simulink model "balancing_sim_model_RL_load_Enes_parallel"  (R2018a)
settings: Solver=ode4  StartTime=0.0  StopTime=Tfinal  FixedStep=Ts  RelTol=1e-3  EnableMultiTasking=on
values from neighbouring files (symbols this model uses):
  Cdc = 15e-6    (= 1.5e-05)    [balancing_sim_parameters.m]
  Cdcrec = 2e-3    (= 0.002)    [balancing_sim_parameters.m]
  delta = 0    [balancing_sim_parameters.m]
  GridFreq = 50    [balancing_sim_parameters.m]
  Lload_1A = 36e-3    (= 0.036)    [balancing_sim_parameters.m]
  Lload_1B = 34e-3    (= 0.034)    [balancing_sim_parameters.m]
  Lload_1C = 36e-3    (= 0.036)    [balancing_sim_parameters.m]
  Lload_2A = 26e-3    (= 0.026)    [balancing_sim_parameters.m]
  Lload_2B = 26e-3    (= 0.026)    [balancing_sim_parameters.m]
  Lload_2C = 26e-3    (= 0.026)    [balancing_sim_parameters.m]
  ma1 = 0.9    [balancing_sim_parameters.m]
  ma2 = 0.9    [balancing_sim_parameters.m]
  phase = [0 90 0 90]    [balancing_sim_parameters.m]
  Rin = 70    [balancing_sim_parameters.m]
  Ripth = 0.08    [balancing_sim_parameters.m]
  Rload_1A = 15.26    [balancing_sim_parameters.m]
  Rload_1B = 15.31    [balancing_sim_parameters.m]
  Rload_1C = 15.26    [balancing_sim_parameters.m]
  Rload_2A = 14.02    [balancing_sim_parameters.m]
  Rload_2B = 14.03    [balancing_sim_parameters.m]
  Rload_2C = 14.00    (= 14)    [balancing_sim_parameters.m]
  Ts = 1e-6    (= 1e-06)    [balancing_sim_parameters.m]
  Vacrms = 230    [balancing_sim_parameters.m]
  Vin = Vdc + Rin*(Pout/Vdc)+3    (= 1061.51851852)    [balancing_sim_parameters.m]
  wout = 2*pi*fout    (= 314.159265359)    [balancing_sim_parameters.m]
undefined symbols (not defined in the file or in its folder): Lload, Rload
libraries: powerlib x45, powerlib_meascontrol x27, simulink x8
settings Model: SimulationMode=accelerator  Creator=ugurm  LastModifiedBy=enes_
settings DataIOCC: LimitDataPoints=on  SaveFormat=Array
settings OptimizationCC: LifeSpan=inf
settings DebuggingCC: UnderspecifiedInitializationDetection=Classic  MergeDetectMultiDrivingBlocksExec=none  SolverPrmCheckMsg=warning  StateNameClashWarn=warning  SFUnexpectedBacktrackingDiag=warning  SFNoUnconditionalDefaultTransitionDiag=warning  SFExecutionAtInitializationDiag=none
settings HardwareCC: ProdBitPerPointer=32  ProdBitPerSizeT=32  ProdBitPerPtrDiffT=32  ProdLargestAtomicFloat=None  ProdIntDivRoundTo=Undefined  ProdEndianess=Unspecified  ProdWordSize=32  ProdHWDeviceType=32-bit Generic
settings ModelReferenceCC: PropagateSignalLabelsOutOfModel=off
settings CodeAppCC: StateflowObjectComments=on
settings GRTTargetCC: TargetLangStandard=C89/C90 (ANSI)  GeneratePreprocessorConditionals=Disable all
settings ConfigComp: CovMetricSettings=dw  CovHtmlReporting=on  CovSaveCumulativeToWorkspaceVar=on  CovSaveSingleToWorkspaceVar=on  CovExternalEMLEnable=off
settings SimscapeCC: SimscapeNormalizeSystem=off

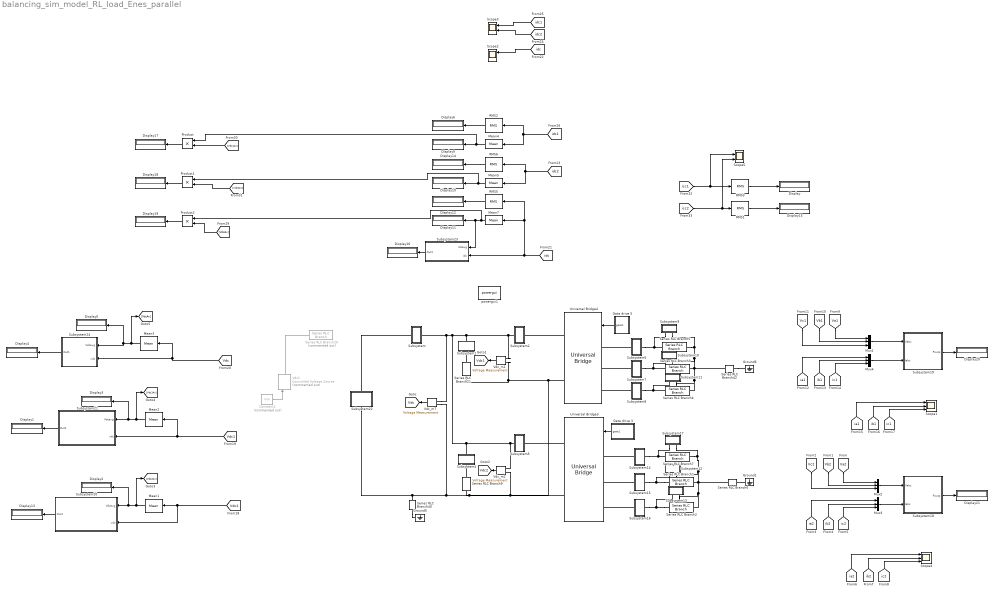
== system balancing_sim_model_RL_load_Enes_parallel ==
  Constant1 : Constant  Commented=on  Value=Vin
  Display{,1..6,9..21} (20 alike) : Display
  Gate drive 3 : Subsystem
  Gate drive 5 : Subsystem
  Ground1 : powerlib/Elements/Ground  LConnTagsString=a
  Ground5 : powerlib/Elements/Ground  LConnTagsString=a
  Ground6 : powerlib/Elements/Ground  LConnTagsString=a
  Mean{1..5,7} (6 alike) : powerlib_meascontrol/Measurements/Mean  Freq=fout  Vinit=0  Ts=0
  Mux{1..4} (4 alike) : Mux  Inputs=3
  Product : Product
  Product1 : Product
  Product2 : Product
  RMS{1..3,5..6} (5 alike) : powerlib_meascontrol/Measurements/RMS  TrueRMS=on  Freq=fout  RMSInit=0  Ts=0
  Scope1 : Scope  NumInputPorts=3
  Scope2 : Scope  NumInputPorts=2
  Scope3 : Scope  NumInputPorts=2
  Scope4 : Scope  NumInputPorts=3
  Scope5 : Scope  NumInputPorts=2
  Series RLC Branch1 : powerlib/Elements/Series RLC Branch  LConnTagsString=__new0  RConnTagsString=__new0  BranchType=RL  Resistance=Rload_2B  Inductance=Lload_2B  SetiL0=off  InitialCurrent=0  Capacitance=1e-6  Setx0=off  InitialVoltage=0  Measurements=None
  Series RLC Branch2 : powerlib/Elements/Series RLC Branch  LConnTagsString=__new0  RConnTagsString=__new0  BranchType=RL  Resistance=Rload_2C  Inductance=Lload_2C  SetiL0=off  InitialCurrent=0  Capacitance=1e-6  Setx0=off  InitialVoltage=0  Measurements=None
  Series RLC Branch20 : powerlib/Elements/Series RLC Branch  Commented=on  LConnTagsString=__new0  RConnTagsString=__new0  BranchType=R  Resistance=Rin  Inductance=1e-3  SetiL0=off  InitialCurrent=0  Capacitance=1e-6  Setx0=off  InitialVoltage=0  Measurements=None
  Series RLC Branch21 : powerlib/Elements/Series RLC Branch  LConnTagsString=__new0  RConnTagsString=__new0  BranchType=C  Resistance=Rload  Inductance=Lload  SetiL0=off  InitialCurrent=0  Capacitance=Cdc  Setx0=off  InitialVoltage=0  Measurements=None
  Series RLC Branch3 : powerlib/Elements/Series RLC Branch  LConnTagsString=__new0  RConnTagsString=__new0  BranchType=RL  Resistance=Rload_1B  Inductance=Lload_1B  SetiL0=off  InitialCurrent=0  Capacitance=1e-6  Setx0=off  InitialVoltage=0  Measurements=None
  Series RLC Branch4 : powerlib/Elements/Series RLC Branch  LConnTagsString=__new0  RConnTagsString=__new0  BranchType=RL  Resistance=Rload_1C  Inductance=Lload_1C  SetiL0=off  InitialCurrent=0  Capacitance=1e-6  Setx0=off  InitialVoltage=0  Measurements=None
  Series RLC Branch40 : powerlib/Elements/Series RLC Branch  LConnTagsString=__new0  RConnTagsString=__new0  BranchType=R  Resistance=1e12  Inductance=Lload  SetiL0=off  InitialCurrent=0  Capacitance=1e-6  Setx0=off  InitialVoltage=0  Measurements=None
  Series RLC Branch42 : powerlib/Elements/Series RLC Branch  LConnTagsString=__new0  RConnTagsString=__new0  BranchType=R  Resistance=1e12  Inductance=Lload  SetiL0=off  InitialCurrent=0  Capacitance=1e-6  Setx0=off  InitialVoltage=0  Measurements=None
  Series RLC Branch5 : powerlib/Elements/Series RLC Branch  LConnTagsString=__new0  RConnTagsString=__new0  BranchType=RL  Resistance=Rload_1A  Inductance=Lload_1A  SetiL0=off  InitialCurrent=0  Capacitance=1e-6  Setx0=off  InitialVoltage=0  Measurements=None
  Series RLC Branch6 : powerlib/Elements/Series RLC Branch  LConnTagsString=__new0  RConnTagsString=__new0  BranchType=R  Resistance=1e12  Inductance=Lload  SetiL0=off  InitialCurrent=0  Capacitance=1e-6  Setx0=off  InitialVoltage=0  Measurements=None
  Series RLC Branch7 : powerlib/Elements/Series RLC Branch  LConnTagsString=__new0  RConnTagsString=__new0  BranchType=RL  Resistance=Rload_2A  Inductance=Lload_2A  SetiL0=off  InitialCurrent=0  Capacitance=1e-6  Setx0=off  InitialVoltage=0  Measurements=None
  Series RLC Branch9 : powerlib/Elements/Series RLC Branch  LConnTagsString=__new0  RConnTagsString=__new0  BranchType=C  Resistance=Rload  Inductance=Lload  SetiL0=off  InitialCurrent=0  Capacitance=Cdc  Setx0=off  InitialVoltage=0  Measurements=None
  Subsystem : Subsystem
  Subsystem1 : Subsystem
  Subsystem10 : Subsystem
  Subsystem11 : Subsystem
  Subsystem12 : Subsystem
  Subsystem13 : Subsystem
  Subsystem14 : Subsystem
  Subsystem15 : Subsystem
  Subsystem16 : Subsystem
  Subsystem17 : Subsystem
  Subsystem18 : Subsystem
  Subsystem19 : Subsystem
  Subsystem2 : Subsystem
  Subsystem20 : Subsystem
  Subsystem21 : Subsystem
  Subsystem22 : Subsystem
  Subsystem23 : Subsystem
  Subsystem24 : Subsystem
  Subsystem4 : Subsystem
  Subsystem5 : Subsystem
  Subsystem6 : Subsystem
  Subsystem7 : Subsystem
  Subsystem8 : Subsystem
  Subsystem9 : Subsystem
  Universal Bridge3 : powerlib/Power Electronics/Universal Bridge  Arms=3  SnubberResistance=1e5  SnubberCapacitance=inf  Device=IGBT / Diodes  Ron=1e-6  Lon=0  ForwardVoltages="[  0  0  ]"  ForwardVoltage=0  GTOparameters=[ 10e-6 , 20e-6 ]  IGBTparameters=[0,0]  Measurements=None  Measurements_2=None  converterType=Rectifier
  Universal Bridge4 : powerlib/Power Electronics/Universal Bridge  Arms=3  SnubberResistance=1e5  SnubberCapacitance=inf  Device=IGBT / Diodes  Ron=1e-6  Lon=0  ForwardVoltages="[  0  0  ]"  ForwardVoltage=0  GTOparameters=[ 10e-6 , 20e-6 ]  IGBTparameters=[0,0]  Measurements=None  Measurements_2=None  converterType=Rectifier
  Vdc1 : powerlib/Electrical Sources/Controlled Voltage Source  Commented=on  Initialize=off  Source_Type=DC  Amplitude=200  Phase=0  Frequency=0  Measurements=None
  Vdc_m1 : powerlib/Measurements/Voltage Measurement  PhasorSimulation=off  OutputType=Complex  PSBequivalent=0
  Vdc_m2 : powerlib/Measurements/Voltage Measurement  PhasorSimulation=off  OutputType=Complex  PSBequivalent=0
  Vdc_m7 : powerlib/Measurements/Voltage Measurement  PhasorSimulation=off  OutputType=Complex  PSBequivalent=0
  powergui1 : powerlib/powergui  Priority=1  SimulationMode=Discrete  SampleTime=Ts  frequency=60  Iterations=50  frequencyindice=0  Pbase=100e6  ErrMax=1e-4  UnitsV=kV  UnitsW=MW  buscounter=0  FunctionMessages=off  echomessages=off  EnableUseOfTLC=off  CurrentSourceSwitches=off  DisableSnubberDevices=off  DisableRonSwitches=off  DisableVfSwitches=off  DisplayEquations=off  SolverType=Tustin  Interpol=off  ExternalGateDelay=off  methode=off  Ts=0  x0status=blocks  SPID=off  SwTol=0  HookPort=off  RestoreLinks=warning  ResistiveCurrentMeasurement=off  Frange=[0:2:500]  Ylog=off  Xlog=on  ShowGrid=off  save=off  variable=ZData  structure=Vdc  ZoomFFT=off  StartTime=0.04  cycles=5  DisplayStyle=5  fundamental=50  FreqAxis=off  MaxFrequency=30000  frequencyindicesteady=1  RmsSteady=1  display=off
  tag scope: Vdc1=global, Vdc2=global, Vdc=global
  wires:
  Constant1/1 -> Vdc1/1
  Vdc_m7/1 -> [Vdc]
  Vdc_m1/1 -> [Vdc1]
  Gate drive 5/1(gate1) -> Universal Bridge4/1
  Vdc_m2/1 -> [Vdc2]
  Gate drive 3/1(gate1) -> Universal Bridge3/1
  Mux3/1 -> Subsystem18/2(Iabc)
  Mux2/1 -> Subsystem18/1(Vabc)
  Subsystem18/1(Poutp) -> Display21/1
  [Va2] -> Mux2/1
  [Vb2] -> Mux2/2
  [Vc2] -> Mux2/3
  [ia2] -> Mux3/1
  [ib2] -> Mux3/2
  [ic2] -> Mux3/3
  [ia2] -> Scope4/1
  [ib2] -> Scope4/2
  [ic2] -> Scope4/3
  Subsystem19/1(Poutp) -> Display20/1
  [ic1] -> Mux4/3
  Mux4/1 -> Subsystem19/2(Iabc)
  Mux1/1 -> Subsystem19/1(Vabc)
  [ia1] -> Mux4/1
  [ib1] -> Mux4/2
  [Va1] -> Mux1/1
  [Vb1] -> Mux1/2
  [Vc1] -> Mux1/3
  [ib1] -> Scope1/2
  [ic1] -> Scope1/3
  [ia1] -> Scope1/1
  Subsystem20/1(Out1) -> Display13/1
  Mean1/1 -> [Vdc2Av], Subsystem20/1(Vdcavg), Display2/1
  [Vdc2] -> Subsystem20/2(vdc), Mean1/1
  Subsystem21/1(Out1) -> Display1/1
  [Vdc1] -> Subsystem21/2(vdc), Mean2/1
  Mean2/1 -> [Vdc1Av], Subsystem21/1(Vdcavg), Display3/1
  Subsystem24/1(Out1) -> Display4/1
  [Vdc] -> Subsystem24/2(vdc), Mean3/1
  RMS2/1 -> Display6/1
  RMS5/1 -> Display12/1
  RMS6/1 -> Display14/1
  Subsystem23/1(Out1) -> Display16/1
  [idc] -> Mean7/1, RMS5/1, Subsystem23/2(idc)
  [idc] -> Scope2/1
  [idc2] -> Mean5/1, RMS6/1
  [idc2] -> Scope3/2
  [idc1] -> Scope3/1
  [idc1] -> RMS2/1, Mean4/1
  Mean7/1 -> Product2/1, Subsystem23/1(Idcavg), Display11/1
  Mean5/1 -> Product1/1, Display10/1
  Product1/1 -> Display18/1
  Product/1 -> Display17/1
  Mean4/1 -> Product/1, Display9/1
  Product2/1 -> Display19/1
  [VdcAv] -> Product2/2
  [Vdc1Av] -> Product/2
  [Vdc2Av] -> Product1/2
  RMS3/1 -> Display/1
  RMS1/1 -> Display15/1
  [icc1] -> Scope5/1, RMS3/1
  [icc2] -> Scope5/2, RMS1/1
  Mean3/1 -> [VdcAv], Subsystem24/1(Vdcavg), Display5/1
  connections:
  Series RLC Branch40/RConn1 -- Ground5/LConn1
  Vdc1/RConn1 -- Series RLC Branch20/LConn1
  Series RLC Branch21/LConn1 -- Subsystem1/LConn1
  Vdc_m2/LConn2 -- Universal Bridge3/RConn2 -- Subsystem22/LConn1 -- Series RLC Branch40/LConn1 -- Vdc_m7/LConn2 -- Universal Bridge4/RConn2 -- Series RLC Branch21/RConn1 -- Vdc_m1/LConn2 -- Series RLC Branch9/RConn1
  Universal Bridge4/RConn1 -- Subsystem2/RConn1
  Series RLC Branch9/LConn1 -- Subsystem4/LConn1
  Vdc_m7/LConn1 -- Vdc_m1/LConn1 -- Subsystem2/LConn1 -- Subsystem1/RConn1 -- Subsystem5/LConn1 -- Vdc_m2/LConn1 -- Subsystem4/RConn1 -- Subsystem/RConn1
  Universal Bridge3/RConn1 -- Subsystem5/RConn1
  Subsystem6/LConn1 -- Universal Bridge4/LConn1
  Subsystem8/LConn1 -- Universal Bridge4/LConn3
  Subsystem7/LConn1 -- Universal Bridge4/LConn2
  Subsystem8/RConn1 -- Subsystem11/LConn1 -- Series RLC Branch4/LConn1
  Subsystem7/RConn1 -- Subsystem10/LConn1 -- Series RLC Branch3/LConn1
  Series RLC Branch5/RConn1 -- Subsystem9/LConn2 -- Subsystem10/LConn2 -- Subsystem11/LConn2 -- Series RLC Branch4/RConn1 -- Series RLC Branch3/RConn1 -- Series RLC Branch42/LConn1
  Series RLC Branch42/RConn1 -- Ground6/LConn1
  Subsystem6/RConn1 -- Subsystem9/LConn1 -- Series RLC Branch5/LConn1
  Series RLC Branch2/RConn1 -- Subsystem13/LConn2 -- Subsystem17/LConn2 -- Series RLC Branch7/RConn1 -- Subsystem12/LConn2 -- Series RLC Branch1/RConn1 -- Series RLC Branch6/LConn1
  Subsystem17/LConn1 -- Series RLC Branch7/LConn1 -- Subsystem14/RConn1
  Series RLC Branch2/LConn1 -- Subsystem13/LConn1 -- Subsystem16/RConn1
  Series RLC Branch1/LConn1 -- Subsystem15/RConn1 -- Subsystem12/LConn1
  Subsystem14/LConn1 -- Universal Bridge3/LConn1
  Subsystem15/LConn1 -- Universal Bridge3/LConn2
  Subsystem16/LConn1 -- Universal Bridge3/LConn3
  Ground1/LConn1 -- Series RLC Branch6/RConn1
  Subsystem22/RConn1 -- Subsystem/LConn1

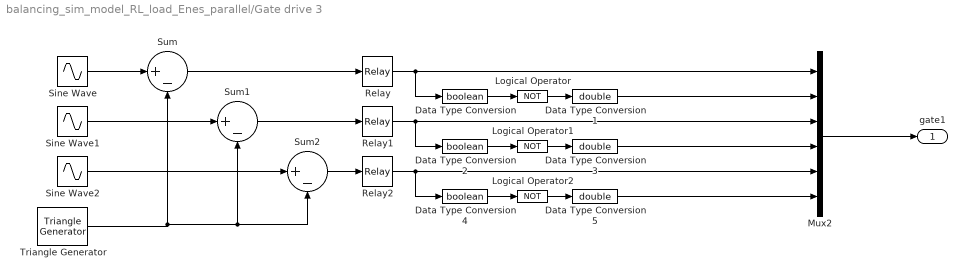
== system balancing_sim_model_RL_load_Enes_parallel/Gate drive 3 ==
  Data Type Conversion : DataTypeConversion  OutDataTypeStr=boolean
  Data Type Conversion1 : DataTypeConversion  OutDataTypeStr=double
  Data Type Conversion2 : DataTypeConversion  OutDataTypeStr=boolean
  Data Type Conversion3 : DataTypeConversion  OutDataTypeStr=double
  Data Type Conversion4 : DataTypeConversion  OutDataTypeStr=boolean
  Data Type Conversion5 : DataTypeConversion  OutDataTypeStr=double
  Logical Operator : Logic  Operator=NOT  AllPortsSameDT=off  OutDataTypeStr=boolean
  Logical Operator1 : Logic  Operator=NOT  AllPortsSameDT=off  OutDataTypeStr=boolean
  Logical Operator2 : Logic  Operator=NOT  AllPortsSameDT=off  OutDataTypeStr=boolean
  Mux2 : Mux  Inputs=6
  Relay : Relay
  Relay1 : Relay
  Relay2 : Relay
  Sine Wave : Sin  Amplitude=ma2  Frequency=wout  Phase=delta  SampleTime=0
  Sine Wave1 : Sin  Amplitude=ma2  Frequency=wout  Phase=-2*pi/3+delta  SampleTime=0
  Sine Wave2 : Sin  Amplitude=ma2  Frequency=wout  Phase=2*pi/3+delta  SampleTime=0
  Sum : Sum  Inputs=|+-
  Sum1 : Sum  Inputs=|+-
  Sum2 : Sum  Inputs=|+-
  Triangle Generator : powerlib_meascontrol/Pulse & Signal Generators/Triangle Generator  Freq=fsw  Phase=phase(3)  Ts=Ts
  gate1 : Outport
  wires:
  Sine Wave/1 -> Sum/1
  Triangle Generator/1 -> Sum1/2, Sum2/2, Sum/2
  Sine Wave1/1 -> Sum1/1
  Sine Wave2/1 -> Sum2/1
  Sum/1 -> Relay/1
  Sum1/1 -> Relay1/1
  Sum2/1 -> Relay2/1
  Data Type Conversion/1 -> Logical Operator/1
  Relay/1 -> Data Type Conversion/1, Mux2/1
  Logical Operator/1 -> Data Type Conversion1/1
  Data Type Conversion1/1 -> Mux2/2
  Data Type Conversion2/1 -> Logical Operator1/1
  Relay1/1 -> Data Type Conversion2/1, Mux2/3
  Logical Operator1/1 -> Data Type Conversion3/1
  Data Type Conversion3/1 -> Mux2/4
  Data Type Conversion4/1 -> Logical Operator2/1
  Relay2/1 -> Data Type Conversion4/1, Mux2/5
  Logical Operator2/1 -> Data Type Conversion5/1
  Data Type Conversion5/1 -> Mux2/6
  Mux2/1 -> gate1/1

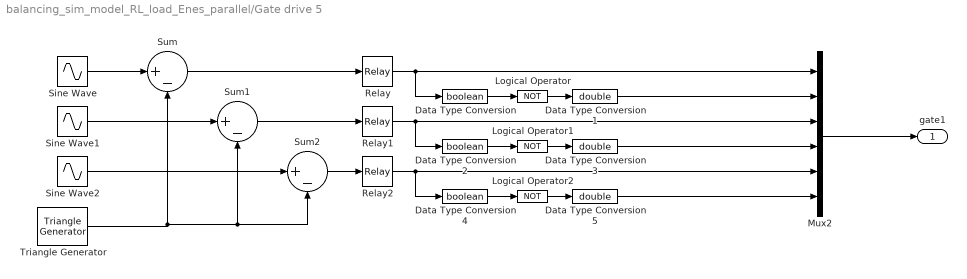
== system balancing_sim_model_RL_load_Enes_parallel/Gate drive 5 ==
  Data Type Conversion : DataTypeConversion  OutDataTypeStr=boolean
  Data Type Conversion1 : DataTypeConversion  OutDataTypeStr=double
  Data Type Conversion2 : DataTypeConversion  OutDataTypeStr=boolean
  Data Type Conversion3 : DataTypeConversion  OutDataTypeStr=double
  Data Type Conversion4 : DataTypeConversion  OutDataTypeStr=boolean
  Data Type Conversion5 : DataTypeConversion  OutDataTypeStr=double
  Logical Operator : Logic  Operator=NOT  AllPortsSameDT=off  OutDataTypeStr=boolean
  Logical Operator1 : Logic  Operator=NOT  AllPortsSameDT=off  OutDataTypeStr=boolean
  Logical Operator2 : Logic  Operator=NOT  AllPortsSameDT=off  OutDataTypeStr=boolean
  Mux2 : Mux  Inputs=6
  Relay : Relay
  Relay1 : Relay
  Relay2 : Relay
  Sine Wave : Sin  Amplitude=ma1  Frequency=wout  Phase=delta  SampleTime=0
  Sine Wave1 : Sin  Amplitude=ma1  Frequency=wout  Phase=-2*pi/3+delta  SampleTime=0
  Sine Wave2 : Sin  Amplitude=ma1  Frequency=wout  Phase=2*pi/3+delta  SampleTime=0
  Sum : Sum  Inputs=|+-
  Sum1 : Sum  Inputs=|+-
  Sum2 : Sum  Inputs=|+-
  Triangle Generator : powerlib_meascontrol/Pulse & Signal Generators/Triangle Generator  Freq=fsw  Phase=phase(1)  Ts=Ts
  gate1 : Outport
  wires:
  Sine Wave/1 -> Sum/1
  Triangle Generator/1 -> Sum1/2, Sum2/2, Sum/2
  Sine Wave1/1 -> Sum1/1
  Sine Wave2/1 -> Sum2/1
  Sum/1 -> Relay/1
  Sum1/1 -> Relay1/1
  Sum2/1 -> Relay2/1
  Data Type Conversion/1 -> Logical Operator/1
  Relay/1 -> Data Type Conversion/1, Mux2/1
  Logical Operator/1 -> Data Type Conversion1/1
  Data Type Conversion1/1 -> Mux2/2
  Data Type Conversion2/1 -> Logical Operator1/1
  Relay1/1 -> Data Type Conversion2/1, Mux2/3
  Logical Operator1/1 -> Data Type Conversion3/1
  Data Type Conversion3/1 -> Mux2/4
  Data Type Conversion4/1 -> Logical Operator2/1
  Relay2/1 -> Data Type Conversion4/1, Mux2/5
  Logical Operator2/1 -> Data Type Conversion5/1
  Data Type Conversion5/1 -> Mux2/6
  Mux2/1 -> gate1/1

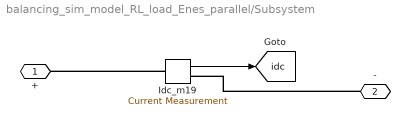
== system balancing_sim_model_RL_load_Enes_parallel/Subsystem ==
  Idc_m19 : powerlib/Measurements/Current Measurement  PhasorSimulation=off  OutputType=Complex  PSBequivalent=0
  + : PMIOPort  Side=Left
  " -" : PMIOPort  Port=2  Side=Right
  tag scope: idc=global
  wires:
  Idc_m19/1 -> [idc]
  connections:
  " -"/RConn1 -- Idc_m19/RConn1
  Idc_m19/LConn1 -- +/RConn1

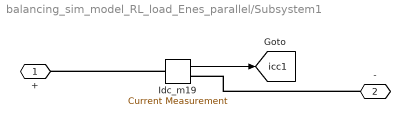
== system balancing_sim_model_RL_load_Enes_parallel/Subsystem1 ==
  Idc_m19 : powerlib/Measurements/Current Measurement  PhasorSimulation=off  OutputType=Complex  PSBequivalent=0
  + : PMIOPort  Side=Left
  " -" : PMIOPort  Port=2  Side=Right
  tag scope: icc1=global
  wires:
  Idc_m19/1 -> [icc1]
  connections:
  " -"/RConn1 -- Idc_m19/RConn1
  Idc_m19/LConn1 -- +/RConn1

== system balancing_sim_model_RL_load_Enes_parallel/Subsystem10 ==
  Vdc_m3 : powerlib/Measurements/Voltage Measurement  PhasorSimulation=off  OutputType=Complex  PSBequivalent=0
  + : PMIOPort  Side=Left
  - : PMIOPort  Port=2  Side=Left
  tag scope: Vb1=global
  wires:
  Vdc_m3/1 -> [Vb1]
  connections:
  Vdc_m3/LConn1 -- +/RConn1
  Vdc_m3/LConn2 -- -/RConn1

== system balancing_sim_model_RL_load_Enes_parallel/Subsystem11 ==
  Vdc_m3 : powerlib/Measurements/Voltage Measurement  PhasorSimulation=off  OutputType=Complex  PSBequivalent=0
  + : PMIOPort  Side=Left
  - : PMIOPort  Port=2  Side=Left
  tag scope: Vc1=global
  wires:
  Vdc_m3/1 -> [Vc1]
  connections:
  Vdc_m3/LConn1 -- +/RConn1
  Vdc_m3/LConn2 -- -/RConn1

== system balancing_sim_model_RL_load_Enes_parallel/Subsystem12 ==
  Vdc_m3 : powerlib/Measurements/Voltage Measurement  PhasorSimulation=off  OutputType=Complex  PSBequivalent=0
  + : PMIOPort  Side=Left
  - : PMIOPort  Port=2  Side=Left
  tag scope: Vb2=global
  wires:
  Vdc_m3/1 -> [Vb2]
  connections:
  Vdc_m3/LConn1 -- +/RConn1
  Vdc_m3/LConn2 -- -/RConn1

== system balancing_sim_model_RL_load_Enes_parallel/Subsystem13 ==
  Vdc_m3 : powerlib/Measurements/Voltage Measurement  PhasorSimulation=off  OutputType=Complex  PSBequivalent=0
  + : PMIOPort  Side=Left
  - : PMIOPort  Port=2  Side=Left
  tag scope: Vc2=global
  wires:
  Vdc_m3/1 -> [Vc2]
  connections:
  Vdc_m3/LConn1 -- +/RConn1
  Vdc_m3/LConn2 -- -/RConn1

== system balancing_sim_model_RL_load_Enes_parallel/Subsystem14 ==
  Idc_m19 : powerlib/Measurements/Current Measurement  PhasorSimulation=off  OutputType=Complex  PSBequivalent=0
  + : PMIOPort  Side=Left
  " -" : PMIOPort  Port=2  Side=Right
  tag scope: ia2=global
  wires:
  Idc_m19/1 -> [ia2]
  connections:
  " -"/RConn1 -- Idc_m19/RConn1
  Idc_m19/LConn1 -- +/RConn1

== system balancing_sim_model_RL_load_Enes_parallel/Subsystem15 ==
  Idc_m19 : powerlib/Measurements/Current Measurement  PhasorSimulation=off  OutputType=Complex  PSBequivalent=0
  + : PMIOPort  Side=Left
  " -" : PMIOPort  Port=2  Side=Right
  tag scope: ib2=global
  wires:
  Idc_m19/1 -> [ib2]
  connections:
  " -"/RConn1 -- Idc_m19/RConn1
  Idc_m19/LConn1 -- +/RConn1

== system balancing_sim_model_RL_load_Enes_parallel/Subsystem16 ==
  Idc_m19 : powerlib/Measurements/Current Measurement  PhasorSimulation=off  OutputType=Complex  PSBequivalent=0
  + : PMIOPort  Side=Left
  " -" : PMIOPort  Port=2  Side=Right
  tag scope: ic2=global
  wires:
  Idc_m19/1 -> [ic2]
  connections:
  " -"/RConn1 -- Idc_m19/RConn1
  Idc_m19/LConn1 -- +/RConn1

== system balancing_sim_model_RL_load_Enes_parallel/Subsystem17 ==
  Vdc_m3 : powerlib/Measurements/Voltage Measurement  PhasorSimulation=off  OutputType=Complex  PSBequivalent=0
  + : PMIOPort  Side=Left
  - : PMIOPort  Port=2  Side=Left
  tag scope: Va2=global
  wires:
  Vdc_m3/1 -> [Va2]
  connections:
  Vdc_m3/LConn1 -- +/RConn1
  Vdc_m3/LConn2 -- -/RConn1

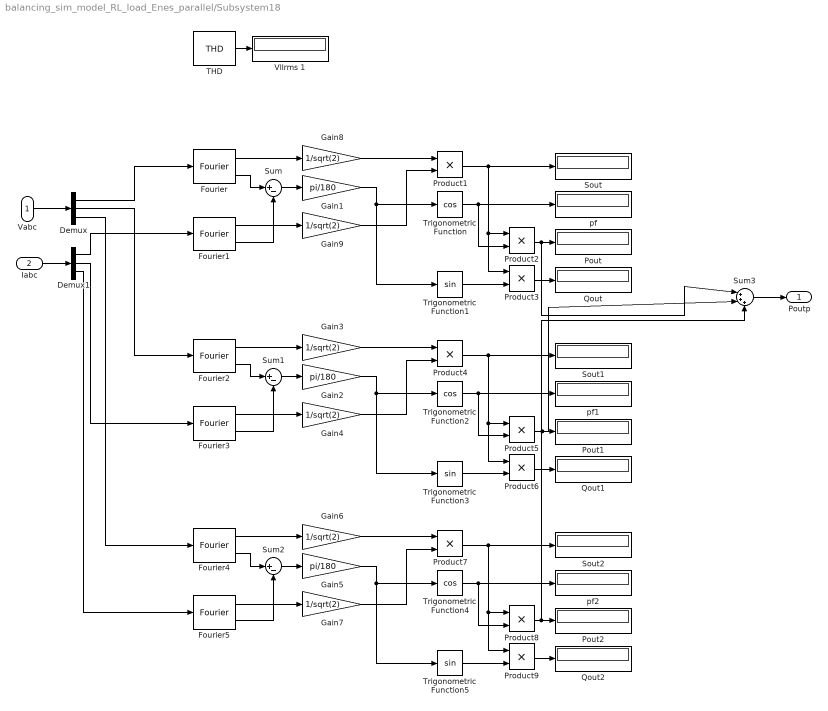
== system balancing_sim_model_RL_load_Enes_parallel/Subsystem18 ==
  Vabc : Inport
  Iabc : Inport  Port=2
  Demux : Demux  Outputs=3
  Demux1 : Demux  Outputs=3
  Fourier{,1..5} (6 alike) : powerlib_meascontrol/Measurements/Fourier  Freq=fout  n=1  InInit=[0, 0]  Ts=Ts
      settings: SourceProductName=Simscape Power Systems
  Gain1 : Gain  Gain=pi/180
  Gain2 : Gain  Gain=pi/180
  Gain{3..4,6..9} (6 alike) : Gain  Gain=1/sqrt(2)
  Gain5 : Gain  Gain=pi/180
  Pout : Display
  Pout1 : Display
  Pout2 : Display
  Product{1..9} (9 alike) : Product
  Qout : Display
  Qout1 : Display
  Qout2 : Display
  Sout : Display
      settings: Format=short_e
  Sout1 : Display
      settings: Format=short_e
  Sout2 : Display
      settings: Format=short_e
  Sum : Sum  Inputs=|+-
  Sum1 : Sum  Inputs=|+-
  Sum2 : Sum  Inputs=|+-
  Sum3 : Sum  Inputs=|+++
  THD : powerlib_meascontrol/Measurements/THD  Freq=fout  Ts=0
  Trigonometric Function : Trigonometry  Operator=cos
  Trigonometric Function1 : Trigonometry
  Trigonometric Function2 : Trigonometry  Operator=cos
  Trigonometric Function3 : Trigonometry
  Trigonometric Function4 : Trigonometry  Operator=cos
  Trigonometric Function5 : Trigonometry
  Vllrms 1 : Display
  pf : Display
  pf1 : Display
  pf2 : Display
  Poutp : Outport
  wires:
  Gain8/1 -> Product1/1
  Gain9/1 -> Product1/2
  Fourier1/1 -> Gain9/1
  Fourier/1 -> Gain8/1
  Product1/1 -> Product3/1, Product2/1, Sout/1
  Sum/1 -> Gain1/1
  Trigonometric Function/1 -> Product2/2, pf/1
  Gain1/1 -> Trigonometric Function1/1, Trigonometric Function/1
  Product2/1 -> Sum3/1, Pout/1
  THD/1 -> Vllrms 1/1
  Vabc/1 -> Demux/1
  Iabc/1 -> Demux1/1
  Fourier/2 -> Sum/1
  Fourier1/2 -> Sum/2
  Trigonometric Function1/1 -> Product3/2
  Product3/1 -> Qout/1
  Gain3/1 -> Product4/1
  Gain4/1 -> Product4/2
  Fourier3/1 -> Gain4/1
  Fourier2/1 -> Gain3/1
  Product4/1 -> Product6/1, Product5/1, Sout1/1
  Sum1/1 -> Gain2/1
  Trigonometric Function2/1 -> Product5/2, pf1/1
  Gain2/1 -> Trigonometric Function3/1, Trigonometric Function2/1
  Product5/1 -> Sum3/2, Pout1/1
  Fourier2/2 -> Sum1/1
  Fourier3/2 -> Sum1/2
  Trigonometric Function3/1 -> Product6/2
  Product6/1 -> Qout1/1
  Gain6/1 -> Product7/1
  Gain7/1 -> Product7/2
  Fourier5/1 -> Gain7/1
  Fourier4/1 -> Gain6/1
  Product7/1 -> Product9/1, Product8/1, Sout2/1
  Sum2/1 -> Gain5/1
  Trigonometric Function4/1 -> Product8/2, pf2/1
  Gain5/1 -> Trigonometric Function5/1, Trigonometric Function4/1
  Fourier4/2 -> Sum2/1
  Fourier5/2 -> Sum2/2
  Trigonometric Function5/1 -> Product9/2
  Product9/1 -> Qout2/1
  Product8/1 -> Sum3/3, Pout2/1
  Sum3/1 -> Poutp/1
  Demux/1 -> Fourier/1
  Demux/2 -> Fourier2/1
  Demux/3 -> Fourier4/1
  Demux1/1 -> Fourier1/1
  Demux1/2 -> Fourier3/1
  Demux1/3 -> Fourier5/1

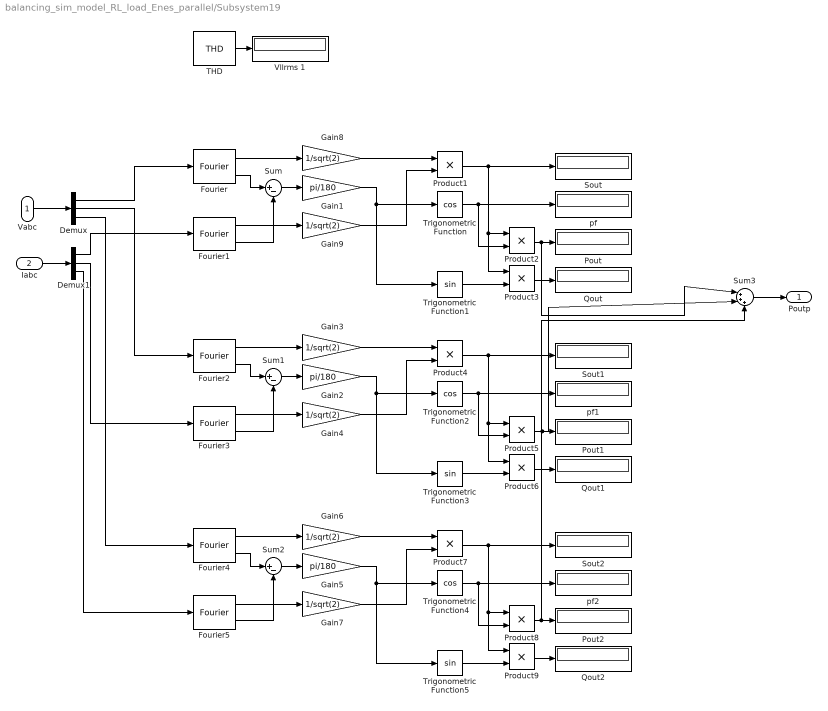
== system balancing_sim_model_RL_load_Enes_parallel/Subsystem19 ==
  Vabc : Inport
  Iabc : Inport  Port=2
  Demux : Demux  Outputs=3
  Demux1 : Demux  Outputs=3
  Fourier{,1..5} (6 alike) : powerlib_meascontrol/Measurements/Fourier  Freq=fout  n=1  InInit=[0, 0]  Ts=Ts
      settings: SourceProductName=Simscape Power Systems
  Gain1 : Gain  Gain=pi/180
  Gain2 : Gain  Gain=pi/180
  Gain{3..4,6..9} (6 alike) : Gain  Gain=1/sqrt(2)
  Gain5 : Gain  Gain=pi/180
  Pout : Display
  Pout1 : Display
  Pout2 : Display
  Product{1..9} (9 alike) : Product
  Qout : Display
  Qout1 : Display
  Qout2 : Display
  Sout : Display
      settings: Format=short_e
  Sout1 : Display
      settings: Format=short_e
  Sout2 : Display
      settings: Format=short_e
  Sum : Sum  Inputs=|+-
  Sum1 : Sum  Inputs=|+-
  Sum2 : Sum  Inputs=|+-
  Sum3 : Sum  Inputs=|+++
  THD : powerlib_meascontrol/Measurements/THD  Freq=fout  Ts=0
  Trigonometric Function : Trigonometry  Operator=cos
  Trigonometric Function1 : Trigonometry
  Trigonometric Function2 : Trigonometry  Operator=cos
  Trigonometric Function3 : Trigonometry
  Trigonometric Function4 : Trigonometry  Operator=cos
  Trigonometric Function5 : Trigonometry
  Vllrms 1 : Display
  pf : Display
  pf1 : Display
  pf2 : Display
  Poutp : Outport
  wires:
  Gain8/1 -> Product1/1
  Gain9/1 -> Product1/2
  Fourier1/1 -> Gain9/1
  Fourier/1 -> Gain8/1
  Product1/1 -> Product3/1, Product2/1, Sout/1
  Sum/1 -> Gain1/1
  Trigonometric Function/1 -> Product2/2, pf/1
  Gain1/1 -> Trigonometric Function1/1, Trigonometric Function/1
  Product2/1 -> Sum3/1, Pout/1
  THD/1 -> Vllrms 1/1
  Vabc/1 -> Demux/1
  Iabc/1 -> Demux1/1
  Fourier/2 -> Sum/1
  Fourier1/2 -> Sum/2
  Trigonometric Function1/1 -> Product3/2
  Product3/1 -> Qout/1
  Gain3/1 -> Product4/1
  Gain4/1 -> Product4/2
  Fourier3/1 -> Gain4/1
  Fourier2/1 -> Gain3/1
  Product4/1 -> Product6/1, Product5/1, Sout1/1
  Sum1/1 -> Gain2/1
  Trigonometric Function2/1 -> Product5/2, pf1/1
  Gain2/1 -> Trigonometric Function3/1, Trigonometric Function2/1
  Product5/1 -> Sum3/2, Pout1/1
  Fourier2/2 -> Sum1/1
  Fourier3/2 -> Sum1/2
  Trigonometric Function3/1 -> Product6/2
  Product6/1 -> Qout1/1
  Gain6/1 -> Product7/1
  Gain7/1 -> Product7/2
  Fourier5/1 -> Gain7/1
  Fourier4/1 -> Gain6/1
  Product7/1 -> Product9/1, Product8/1, Sout2/1
  Sum2/1 -> Gain5/1
  Trigonometric Function4/1 -> Product8/2, pf2/1
  Gain5/1 -> Trigonometric Function5/1, Trigonometric Function4/1
  Fourier4/2 -> Sum2/1
  Fourier5/2 -> Sum2/2
  Trigonometric Function5/1 -> Product9/2
  Product9/1 -> Qout2/1
  Product8/1 -> Sum3/3, Pout2/1
  Sum3/1 -> Poutp/1
  Demux/1 -> Fourier/1
  Demux/2 -> Fourier2/1
  Demux/3 -> Fourier4/1
  Demux1/1 -> Fourier1/1
  Demux1/2 -> Fourier3/1
  Demux1/3 -> Fourier5/1

== system balancing_sim_model_RL_load_Enes_parallel/Subsystem2 ==
  Idc_m19 : powerlib/Measurements/Current Measurement  PhasorSimulation=off  OutputType=Complex  PSBequivalent=0
  + : PMIOPort  Side=Left
  " -" : PMIOPort  Port=2  Side=Right
  tag scope: idc1=global
  wires:
  Idc_m19/1 -> [idc1]
  connections:
  " -"/RConn1 -- Idc_m19/RConn1
  Idc_m19/LConn1 -- +/RConn1

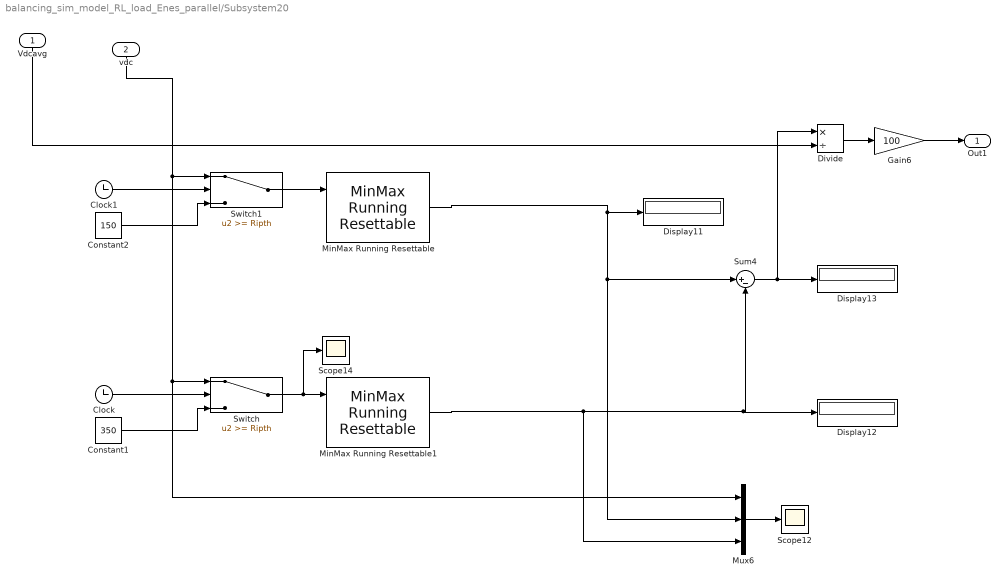
== system balancing_sim_model_RL_load_Enes_parallel/Subsystem20 ==
  Vdcavg : Inport
  vdc : Inport  Port=2
  Clock : Clock
  Clock1 : Clock
  Constant1 : Constant  Value=350  SampleTime=Ts
  Constant2 : Constant  Value=150  SampleTime=Ts
  Display11 : Display
  Display12 : Display
  Display13 : Display
  Divide : Product  Inputs=*/
  Gain6 : Gain  Gain=100
  MinMax Running Resettable : simulink/Math Operations/MinMax Running Resettable  Function=max  vinit=0.0
  MinMax Running Resettable1 : simulink/Math Operations/MinMax Running Resettable  Function=min  vinit=700
  Mux6 : Mux  Inputs=3
  Scope12 : Scope
  Scope14 : Scope
  Sum4 : Sum  Inputs=|+-
  Switch : Switch  Threshold=Ripth
  Switch1 : Switch  Threshold=Ripth
  Out1 : Outport
  wires:
  MinMax Running Resettable/1 -> Display11/1, Mux6/2, Sum4/1
  Clock/1 -> Switch/2
  Gain6/1 -> Out1/1
  Constant1/1 -> Switch/3
  MinMax Running Resettable1/1 -> Mux6/3, Display12/1, Sum4/2
  Switch/1 -> Scope14/1, MinMax Running Resettable1/1
  Sum4/1 -> Divide/1, Display13/1
  Divide/1 -> Gain6/1
  Mux6/1 -> Scope12/1
  Vdcavg/1 -> Divide/2
  vdc/1 -> Switch1/1, Mux6/1, Switch/1
  Switch1/1 -> MinMax Running Resettable/1
  Clock1/1 -> Switch1/2
  Constant2/1 -> Switch1/3

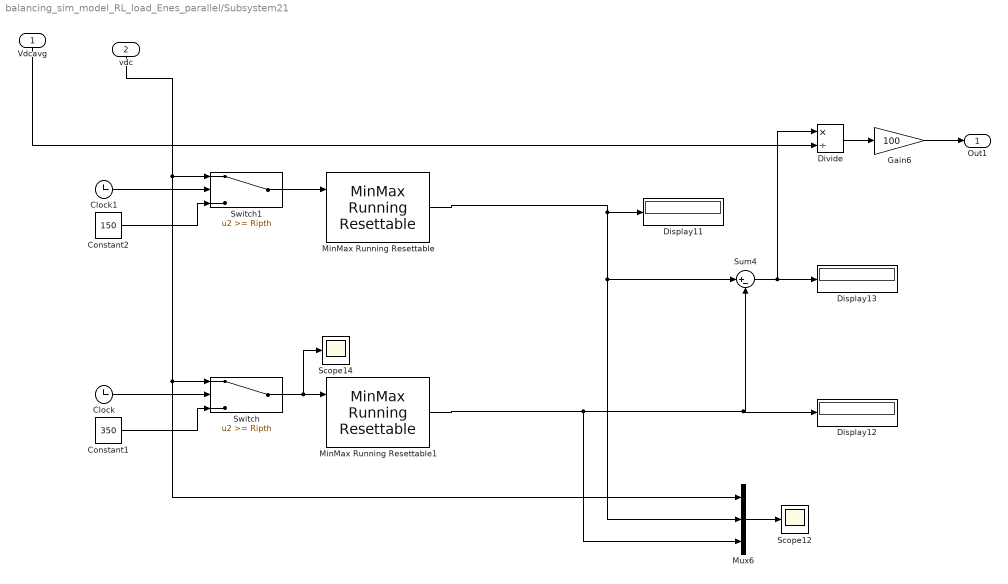
== system balancing_sim_model_RL_load_Enes_parallel/Subsystem21 ==
  Vdcavg : Inport
  vdc : Inport  Port=2
  Clock : Clock
  Clock1 : Clock
  Constant1 : Constant  Value=350  SampleTime=Ts
  Constant2 : Constant  Value=150  SampleTime=Ts
  Display11 : Display
  Display12 : Display
  Display13 : Display
  Divide : Product  Inputs=*/
  Gain6 : Gain  Gain=100
  MinMax Running Resettable : simulink/Math Operations/MinMax Running Resettable  Function=max  vinit=0.0
  MinMax Running Resettable1 : simulink/Math Operations/MinMax Running Resettable  Function=min  vinit=700
  Mux6 : Mux  Inputs=3
  Scope12 : Scope
  Scope14 : Scope
  Sum4 : Sum  Inputs=|+-
  Switch : Switch  Threshold=Ripth
  Switch1 : Switch  Threshold=Ripth
  Out1 : Outport
  wires:
  MinMax Running Resettable/1 -> Display11/1, Mux6/2, Sum4/1
  Clock/1 -> Switch/2
  Gain6/1 -> Out1/1
  Constant1/1 -> Switch/3
  MinMax Running Resettable1/1 -> Mux6/3, Display12/1, Sum4/2
  Switch/1 -> Scope14/1, MinMax Running Resettable1/1
  Sum4/1 -> Divide/1, Display13/1
  Divide/1 -> Gain6/1
  Mux6/1 -> Scope12/1
  Vdcavg/1 -> Divide/2
  vdc/1 -> Switch1/1, Mux6/1, Switch/1
  Switch1/1 -> MinMax Running Resettable/1
  Clock1/1 -> Switch1/2
  Constant2/1 -> Switch1/3

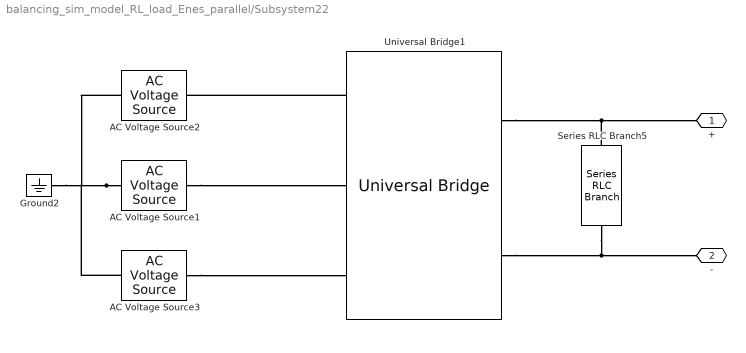
== system balancing_sim_model_RL_load_Enes_parallel/Subsystem22 ==
  AC Voltage Source1 : powerlib/Electrical Sources/AC Voltage Source  Amplitude=Vacrms*sqrt(2)  Phase=-120  Frequency=GridFreq  SampleTime=0  Measurements=None  BusType=swing  Pref=10e3  Qref=0  Qmin=-inf  Qmax=+inf
  AC Voltage Source2 : powerlib/Electrical Sources/AC Voltage Source  Amplitude=Vacrms*sqrt(2)  Phase=0  Frequency=GridFreq  SampleTime=0  Measurements=None  BusType=swing  Pref=10e3  Qref=0  Qmin=-inf  Qmax=+inf
  AC Voltage Source3 : powerlib/Electrical Sources/AC Voltage Source  Amplitude=Vacrms*sqrt(2)  Phase=-240  Frequency=GridFreq  SampleTime=0  Measurements=None  BusType=swing  Pref=10e3  Qref=0  Qmin=-inf  Qmax=+inf
  Ground2 : powerlib/Elements/Ground  LConnTagsString=a
  Series RLC Branch5 : powerlib/Elements/Series RLC Branch  LConnTagsString=__new0  RConnTagsString=__new0  BranchType=C  Resistance=Rload  Inductance=Lload  SetiL0=off  InitialCurrent=0  Capacitance=Cdcrec  Setx0=on  InitialVoltage=270  Measurements=None
  Universal Bridge1 : powerlib/Power Electronics/Universal Bridge  Arms=3  SnubberResistance=1e5  SnubberCapacitance=inf  Device=Diodes  Ron=1e-6  Lon=0  ForwardVoltages="[  0  0  ]"  ForwardVoltage=0  GTOparameters=[ 10e-6 , 20e-6 ]  IGBTparameters=[0,0]  Measurements=None  Measurements_2=None  converterType=Rectifier
  + : PMIOPort  Side=Right
  - : PMIOPort  Port=2  Side=Left
  connections:
  Universal Bridge1/RConn1 -- Series RLC Branch5/LConn1 -- +/RConn1
  Universal Bridge1/RConn2 -- Series RLC Branch5/RConn1 -- -/RConn1
  AC Voltage Source3/RConn1 -- Universal Bridge1/LConn3
  AC Voltage Source1/LConn1 -- Ground2/LConn1 -- AC Voltage Source3/LConn1 -- AC Voltage Source2/LConn1
  AC Voltage Source1/RConn1 -- Universal Bridge1/LConn2
  Universal Bridge1/LConn1 -- AC Voltage Source2/RConn1

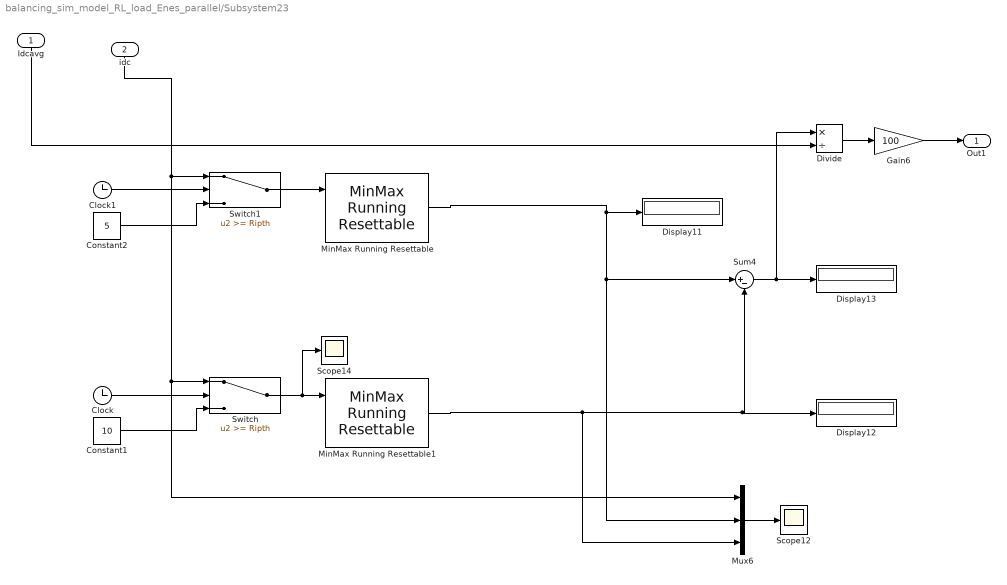
== system balancing_sim_model_RL_load_Enes_parallel/Subsystem23 ==
  Idcavg : Inport
  idc : Inport  Port=2
  Clock : Clock
  Clock1 : Clock
  Constant1 : Constant  Value=10  SampleTime=Ts
  Constant2 : Constant  Value=5  SampleTime=Ts
  Display11 : Display
  Display12 : Display
  Display13 : Display
  Divide : Product  Inputs=*/
  Gain6 : Gain  Gain=100
  MinMax Running Resettable : simulink/Math Operations/MinMax Running Resettable  Function=max  vinit=0.0
  MinMax Running Resettable1 : simulink/Math Operations/MinMax Running Resettable  Function=min  vinit=700
  Mux6 : Mux  Inputs=3
  Scope12 : Scope
  Scope14 : Scope
  Sum4 : Sum  Inputs=|+-
  Switch : Switch  Threshold=Ripth
  Switch1 : Switch  Threshold=Ripth
  Out1 : Outport
  wires:
  MinMax Running Resettable/1 -> Display11/1, Mux6/2, Sum4/1
  Clock/1 -> Switch/2
  Gain6/1 -> Out1/1
  Constant1/1 -> Switch/3
  MinMax Running Resettable1/1 -> Mux6/3, Display12/1, Sum4/2
  Switch/1 -> Scope14/1, MinMax Running Resettable1/1
  Sum4/1 -> Divide/1, Display13/1
  Divide/1 -> Gain6/1
  Mux6/1 -> Scope12/1
  Idcavg/1 -> Divide/2
  idc/1 -> Switch1/1, Mux6/1, Switch/1
  Switch1/1 -> MinMax Running Resettable/1
  Clock1/1 -> Switch1/2
  Constant2/1 -> Switch1/3

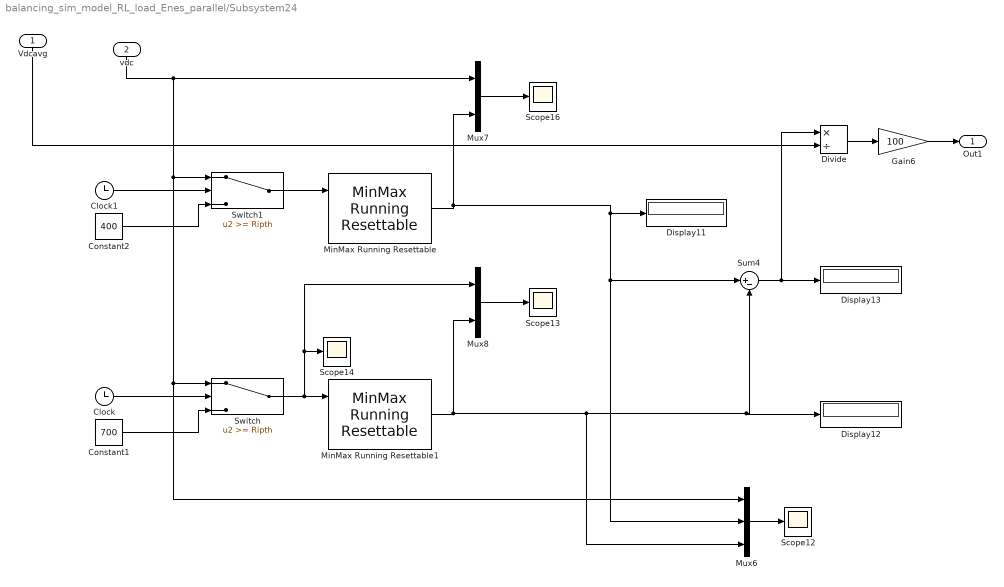
== system balancing_sim_model_RL_load_Enes_parallel/Subsystem24 ==
  Vdcavg : Inport
  vdc : Inport  Port=2
  Clock : Clock
  Clock1 : Clock
  Constant1 : Constant  Value=700  SampleTime=Ts
  Constant2 : Constant  Value=400  SampleTime=Ts
  Display11 : Display
  Display12 : Display
  Display13 : Display
  Divide : Product  Inputs=*/
  Gain6 : Gain  Gain=100
  MinMax Running Resettable : simulink/Math Operations/MinMax Running Resettable  Function=max  vinit=0.0
  MinMax Running Resettable1 : simulink/Math Operations/MinMax Running Resettable  Function=min  vinit=700
  Mux6 : Mux  Inputs=3
  Mux7 : Mux  Inputs=2
  Mux8 : Mux  Inputs=2
  Scope{12..14,16} (4 alike) : Scope
  Sum4 : Sum  Inputs=|+-
  Switch : Switch  Threshold=Ripth
  Switch1 : Switch  Threshold=Ripth
  Out1 : Outport
  wires:
  MinMax Running Resettable/1 -> Display11/1, Mux6/2, Sum4/1, Mux7/2
  Clock/1 -> Switch/2
  Mux8/1 -> Scope13/1
  Gain6/1 -> Out1/1
  Constant1/1 -> Switch/3
  MinMax Running Resettable1/1 -> Mux6/3, Display12/1, Sum4/2, Mux8/2
  Mux7/1 -> Scope16/1
  Switch/1 -> Mux8/1, Scope14/1, MinMax Running Resettable1/1
  Sum4/1 -> Divide/1, Display13/1
  Divide/1 -> Gain6/1
  Mux6/1 -> Scope12/1
  Vdcavg/1 -> Divide/2
  vdc/1 -> Mux7/1, Switch1/1, Mux6/1, Switch/1
  Switch1/1 -> MinMax Running Resettable/1
  Clock1/1 -> Switch1/2
  Constant2/1 -> Switch1/3

== system balancing_sim_model_RL_load_Enes_parallel/Subsystem4 ==
  Idc_m19 : powerlib/Measurements/Current Measurement  PhasorSimulation=off  OutputType=Complex  PSBequivalent=0
  + : PMIOPort  Side=Left
  " -" : PMIOPort  Port=2  Side=Right
  tag scope: icc2=global
  wires:
  Idc_m19/1 -> [icc2]
  connections:
  " -"/RConn1 -- Idc_m19/RConn1
  Idc_m19/LConn1 -- +/RConn1

== system balancing_sim_model_RL_load_Enes_parallel/Subsystem5 ==
  Idc_m19 : powerlib/Measurements/Current Measurement  PhasorSimulation=off  OutputType=Complex  PSBequivalent=0
  + : PMIOPort  Side=Left
  " -" : PMIOPort  Port=2  Side=Right
  tag scope: idc2=global
  wires:
  Idc_m19/1 -> [idc2]
  connections:
  " -"/RConn1 -- Idc_m19/RConn1
  Idc_m19/LConn1 -- +/RConn1

== system balancing_sim_model_RL_load_Enes_parallel/Subsystem6 ==
  Idc_m19 : powerlib/Measurements/Current Measurement  PhasorSimulation=off  OutputType=Complex  PSBequivalent=0
  + : PMIOPort  Side=Left
  " -" : PMIOPort  Port=2  Side=Right
  tag scope: ia1=global
  wires:
  Idc_m19/1 -> [ia1]
  connections:
  " -"/RConn1 -- Idc_m19/RConn1
  Idc_m19/LConn1 -- +/RConn1

== system balancing_sim_model_RL_load_Enes_parallel/Subsystem7 ==
  Idc_m19 : powerlib/Measurements/Current Measurement  PhasorSimulation=off  OutputType=Complex  PSBequivalent=0
  + : PMIOPort  Side=Left
  " -" : PMIOPort  Port=2  Side=Right
  tag scope: ib1=global
  wires:
  Idc_m19/1 -> [ib1]
  connections:
  " -"/RConn1 -- Idc_m19/RConn1
  Idc_m19/LConn1 -- +/RConn1

== system balancing_sim_model_RL_load_Enes_parallel/Subsystem8 ==
  Idc_m19 : powerlib/Measurements/Current Measurement  PhasorSimulation=off  OutputType=Complex  PSBequivalent=0
  + : PMIOPort  Side=Left
  " -" : PMIOPort  Port=2  Side=Right
  tag scope: ic1=global
  wires:
  Idc_m19/1 -> [ic1]
  connections:
  " -"/RConn1 -- Idc_m19/RConn1
  Idc_m19/LConn1 -- +/RConn1

== system balancing_sim_model_RL_load_Enes_parallel/Subsystem9 ==
  Vdc_m3 : powerlib/Measurements/Voltage Measurement  PhasorSimulation=off  OutputType=Complex  PSBequivalent=0
  + : PMIOPort  Side=Left
  - : PMIOPort  Port=2  Side=Left
  tag scope: Va1=global
  wires:
  Vdc_m3/1 -> [Va1]
  connections:
  Vdc_m3/LConn1 -- +/RConn1
  Vdc_m3/LConn2 -- -/RConn1
